simulink model "sampleModel2020_2_sub"  (R2023a)
settings: Solver=VariableStepAuto  StartTime=0.0  StopTime=10.0  RelTol=1e-3
libraries: hdlsllib x8, simulink x2
settings Model: Creator=user1  LastModifiedBy=user1

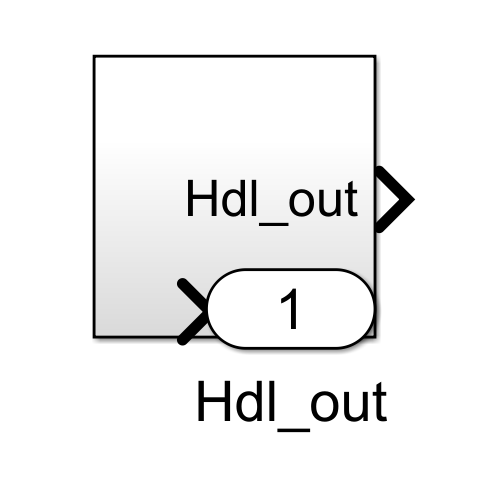
[thumbnail: Simulink's stored preview of the top-level diagram]
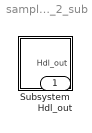
== system sampleModel2020_2_sub ==
  Subsystem : Subsystem
  Hdl_out : Outport  OutDataTypeStr=uint8

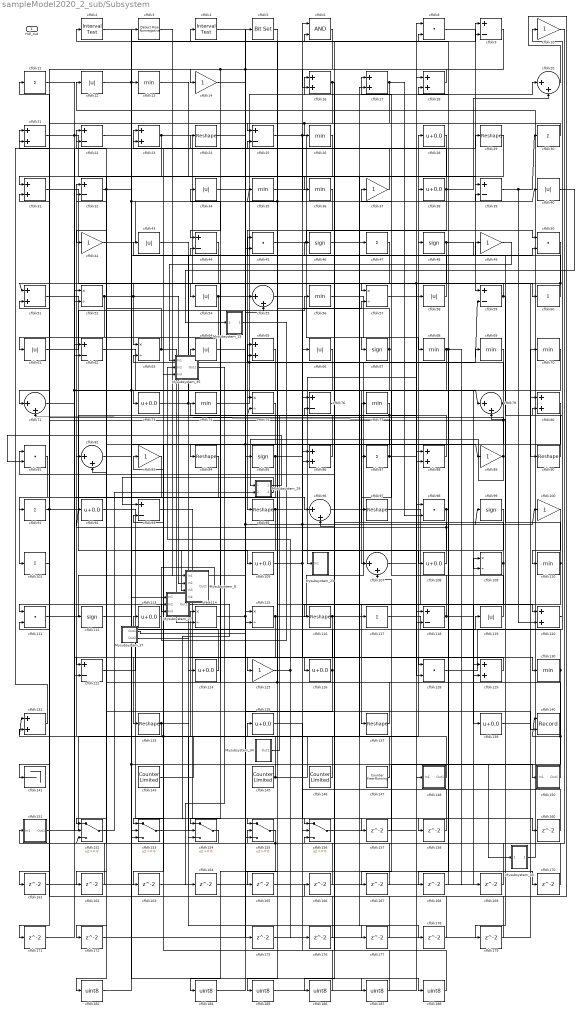
== system sampleModel2020_2_sub/Subsystem ==
  Mysubsystem_15 : Subsystem  TreatAsAtomicUnit=on  RTWFcnName=Mysubsystem_15
      settings: RTWFcnNameOpts=User specified  RTWFileNameOpts=Use function name
  Mysubsystem_23 : Subsystem  TreatAsAtomicUnit=on  RTWFcnName=Mysubsystem_23
      settings: RTWFcnNameOpts=User specified  RTWFileNameOpts=Use function name
  Mysubsystem_27 : Subsystem  TreatAsAtomicUnit=on  RTWFcnName=Mysubsystem_27
      settings: RTWFcnNameOpts=User specified  RTWFileNameOpts=Use function name
  Mysubsystem_29 : Subsystem  TreatAsAtomicUnit=on  RTWFcnName=Mysubsystem_29
      settings: RTWFcnNameOpts=User specified  RTWFileNameOpts=Use function name
  Mysubsystem_34 : Subsystem  TreatAsAtomicUnit=on  RTWFcnName=Mysubsystem_34
      settings: RTWFcnNameOpts=User specified  RTWFileNameOpts=Use function name
  Mysubsystem_35 : Subsystem  TreatAsAtomicUnit=on  RTWFcnName=Mysubsystem_35
      settings: RTWFcnNameOpts=User specified  RTWFileNameOpts=Use function name
  Mysubsystem_37 : Subsystem  TreatAsAtomicUnit=on  RTWFcnName=Mysubsystem_37
      settings: RTWFcnNameOpts=User specified  RTWFileNameOpts=Use function name
  Mysubsystem_43 : Subsystem  TreatAsAtomicUnit=on  RTWFcnName=Mysubsystem_43
      settings: RTWFcnNameOpts=User specified  RTWFileNameOpts=Use function name
  Mysubsystem_8 : Subsystem  TreatAsAtomicUnit=on  RTWFcnName=Mysubsystem_8
      settings: RTWFcnNameOpts=User specified  RTWFileNameOpts=Use function name
  cfblk{10,14,37,42,49,83,89,100,125} (9 alike) : Gain  OutDataTypeStr=uint8
  cfblk{11,30,47,60,87,91,101,117} (8 alike) : Sum  Inputs=+  OutDataTypeStr=uint8
  cfblk{28,38,73,92,105,108,113,124,126,135,139} (11 alike) : Bias  Bias=0.0  SaturateOnIntegerOverflow=off
  cfblk{20,55,71,79,82,96,107} (7 alike) : Sum  Inputs=|++  OutDataTypeStr=uint8
  cfblk{52,57,63,75,109,114..115} (7 alike) : Product  Inputs=*/  OutDataTypeStr=uint8  RndMeth=Zero  SaturateOnIntegerOverflow=on
  cfblk{13,26,35..36,56,68..70,74,77,110,130} (12 alike) : MinMax  OutDataTypeStr=uint8
  cfblk{8,45,50,81,98,111,128} (7 alike) : DotProduct  OutDataTypeStr=uint8
  cfblk{46,48,67,85,99,112} (6 alike) : Signum
  cfblk{24,29,84,90,95,97,116,133,137} (9 alike) : Reshape
  cfblk{9,22,25,32,39,44,59,62,76,93,118,122} (12 alike) : Sum  Inputs=+-  OutDataTypeStr=uint8
  cfblk{12,34,40,43,54,58,61,64,66,119} (10 alike) : Abs  OutDataTypeStr=uint8  SaturateOnIntegerOverflow=off
  cfblk{16..18,21,23,31,51,65,80,86,88,120,129,131} (14 alike) : Sum  OutDataTypeStr=uint8
  cfblk140 : Record  FileSettingsInternal="{\"entries\":[{\"content\":{\"excelSettings\":{\"content\":{},\"type\":\"Streamout.ExcelSettings\"}},\"type\":\"Streamout.FileSettingStorage\",\"uuid\":\"\"}],\"packageUris\":[\"http:\\/\\/schema.mathworks.com\\/mf0\\/streamout_blocks\\/R2020a\"],\"version\":\"1.0\"}"  Layout=[1 1]  SignalsInternal="{\"entries\":[{\"content\":{\"signals\":[{\"content\":{\"blockPath\":[],\"dimensions\":[1],\"domain\":\"\",\"lineColor\":\"#a2142f\",\"plots\":[1],\"port\":1,\"signalID\":59444,\"signalName\":\"cfblk150\"},\"type\":\"RecordBlkView.Signal\",\"uuid\":\"\"},{\"content\":{\"blockPath\":[],\"dimensions\":[1],\"domain\":\"\",\"lineColor\":\"#139fff\",\"plots\":[1],\"port\":2,\"signalID\":59447,\"signalName\":\"cfblk54\"},\"type\":\"RecordBlkView.Signal\",\"uuid\":\"\"}]},\"type\":\"RecordBlkView.InputSignals\",\"uuid\":\"\"}],\"packageUris\":[\"http:\\/\\/schema.mathworks.com\\/mf0\\/streamout_blocks\\/R2020a\"],\"version\":\"1.0\"}"  VisualizationBindings="{\"xyplotplugin\":{\"info\":[{\"series\":[{\"bindingParametersList\":[{\"parameter\":\"X-Axis\",\"signalID\":59444,\"signalName\":\"cfblk150\"},{\"parameter\":\"Y-Axis\",\"signalID\":59447,\"signalName\":\"cfblk54\"}],\"seriesID\":10474}],\"subplotID\":1}]}}"  CompatibilityTag=XY  st=-1
  cfblk141 : Terminator
  cfblk143 : hdlsllib/Sources/Counter Limited  uplimit=7  tsamp=-1
  cfblk145 : hdlsllib/Sources/Counter Limited  uplimit=7  tsamp=-1
  cfblk146 : hdlsllib/Sources/Counter Limited  uplimit=7  tsamp=-1
  cfblk147 : hdlsllib/Sources/Counter Free-Running  NumBits=16  tsamp=-1
  cfblk148 : Subsystem
      settings: LibrarySourceBlock=|
      | hdlsllib/Ports &
      | Subsystems/Subsystem
  cfblk150 : Subsystem
      settings: LibrarySourceBlock=|
      | hdlsllib/Ports &
      | Subsystems/Subsystem
  cfblk151 : Subsystem
      settings: LibrarySourceBlock=|
      | hdlsllib/Ports &
      | Subsystems/Subsystem
  cfblk{152..156} (5 alike) : Switch  OutDataTypeStr=uint8  SaturateOnIntegerOverflow=off  InputSameDT=off
  cfblk{157..158,160..172,175..179} (20 alike) : Delay  SampleTime=1
  cfblk{182,184..188} (6 alike) : DataTypeConversion  OutDataTypeStr=uint8  SaturateOnIntegerOverflow=off  RndMeth=Floor
  cfblk2 : hdlsllib/Logic and Bit Operations/Interval Test  IntervalClosedRight=on  uplimit=0.5  IntervalClosedLeft=on  lowlimit=-0.5  OutDataTypeStr=uint8
  cfblk3 : hdlsllib/Logic and Bit Operations/Detect Rise Nonnegative  vinit=0  OutDataTypeStr=uint8
  cfblk4 : hdlsllib/Logic and Bit Operations/Interval Test  IntervalClosedRight=on  uplimit=0.5  IntervalClosedLeft=on  lowlimit=-0.5  OutDataTypeStr=uint8
  cfblk5 : simulink/Logic and Bit Operations/Bit Set  iBit=0
      settings: LibrarySourceBlock=|
      | hdlsllib/Logic and Bit
      | Operations/Bit Set
  cfblk6 : Logic  AllPortsSameDT=off  OutDataTypeStr=boolean
  Hdl_out : Outport  OutDataTypeStr=uint8
  wires:
  cfblk28/1 -> cfblk31/1
  cfblk66/1 -> cfblk73/1
  cfblk44/1 -> cfblk63/1, Mysubsystem_8/2(In2)
  cfblk100/1 -> cfblk110/1
  cfblk109/1 -> cfblk81/1, cfblk137/1
  cfblk25/1 -> cfblk130/1, cfblk67/1
  cfblk98/1 -> cfblk153/3, cfblk2/1
  cfblk93/1 -> cfblk156/1
  cfblk16/1 -> cfblk126/1, cfblk125/1, cfblk26/1
  cfblk145/1 -> cfblk111/2, cfblk28/1
  cfblk150/1(Out1) -> cfblk44/2, cfblk140/1
  cfblk124/1 -> cfblk83/1
  cfblk113/1 -> cfblk111/1
  cfblk115/1 -> cfblk122/2, cfblk38/1
  cfblk146/1 -> cfblk32/1
  cfblk59/1 -> cfblk179/1, cfblk54/1
  cfblk95/1 -> cfblk120/1, Mysubsystem_8/3(In3)
  cfblk88/1 -> cfblk17/1
  cfblk56/1 -> cfblk88/2
  cfblk155/1 -> cfblk184/1, cfblk152/3
  cfblk35/1 -> cfblk68/1
  cfblk110/1 -> cfblk165/1, cfblk79/2
  cfblk51/1 -> cfblk105/1
  cfblk84/1 -> cfblk153/1
  cfblk99/1 -> cfblk116/1
  cfblk131/1 -> cfblk22/1
  cfblk70/1 -> cfblk107/1
  cfblk32/1 -> cfblk188/1, cfblk162/1
  cfblk54/1 -> cfblk140/2, cfblk61/1
  cfblk128/1 -> cfblk80/2
  cfblk23/1 -> cfblk82/2, cfblk90/1
  cfblk117/1 -> cfblk119/1
  cfblk62/1 -> cfblk109/2
  cfblk105/1 -> cfblk118/2, cfblk57/2, cfblk99/1
  cfblk74/1 -> cfblk59/2, cfblk16/1
  cfblk45/1 -> cfblk50/1, cfblk60/1
  cfblk18/1 -> cfblk14/1
  cfblk26/1 -> cfblk52/2
  cfblk147/1 -> cfblk114/1
  cfblk61/1 -> cfblk56/1
  cfblk37/1 -> cfblk23/1
  cfblk34/1 -> cfblk20/1
  cfblk92/1 -> cfblk155/1
  cfblk82/1 -> cfblk48/1
  cfblk36/1 -> cfblk95/1
  cfblk156/1 -> cfblk8/1
  cfblk10/1 -> cfblk155/2
  cfblk22/1 -> cfblk3/1
  cfblk21/1 -> cfblk96/1, cfblk117/1
  cfblk154/1 -> cfblk151/1(In1)
  cfblk24/1 -> cfblk160/1, cfblk89/1
  cfblk151/1(Out1) -> cfblk47/1
  cfblk116/1 -> cfblk178/1, cfblk133/1
  cfblk67/1 -> cfblk4/1, cfblk154/1
  cfblk60/1 -> cfblk46/1, cfblk51/1
  cfblk17/1 -> cfblk98/2, cfblk141/1
  cfblk39/1 -> cfblk120/2, cfblk30/1
  cfblk126/1 -> cfblk152/1, cfblk64/1
  cfblk77/1 -> cfblk182/1, cfblk75/2
  cfblk122/1 -> cfblk55/1
  cfblk79/1 -> cfblk96/2, cfblk34/1
  cfblk125/1 -> cfblk176/1, Mysubsystem_35/2(In2)
  cfblk14/1 -> cfblk57/1
  cfblk31/1 -> cfblk66/1
  cfblk12/1 -> cfblk13/1, cfblk187/1, Mysubsystem_43/1(In1)
  cfblk38/1 -> cfblk75/1, cfblk20/2, cfblk24/1
  cfblk96/1 -> cfblk58/1
  cfblk86/1 -> cfblk45/1
  cfblk52/1 -> cfblk62/2, Mysubsystem_27/1(In1)
  cfblk43/1 -> cfblk124/1
  cfblk8/1 -> cfblk59/1
  cfblk47/1 -> cfblk84/1
  cfblk6/1 -> cfblk155/3, cfblk171/1, cfblk44/1
  cfblk89/1 -> cfblk31/2, cfblk21/1, Mysubsystem_29/1(In1)
  cfblk97/1 -> cfblk129/1
  cfblk139/1 -> cfblk70/1
  cfblk85/1 -> cfblk87/1, cfblk101/1
  cfblk91/1 -> cfblk21/2, cfblk18/1
  cfblk130/1 -> cfblk167/1, cfblk65/1
  cfblk48/1 -> cfblk50/2, cfblk71/1, Mysubsystem_23/1(In1)
  cfblk120/1 -> cfblk10/1
  cfblk69/1 -> cfblk128/1
  cfblk118/1 -> cfblk63/2, cfblk139/1
  cfblk4/1 -> cfblk36/1
  cfblk13/1 -> cfblk39/1
  cfblk111/1 -> cfblk55/2
  cfblk65/1 -> cfblk152/2, cfblk153/2
  cfblk68/1 -> cfblk97/1, cfblk169/1, cfblk168/1
  cfblk108/1 -> cfblk92/1, cfblk77/1
  cfblk148/1(Out1) -> cfblk131/1, Mysubsystem_35/3(In3)
  cfblk101/1 -> cfblk11/1
  cfblk133/1 -> cfblk177/1, cfblk131/2
  cfblk55/1 -> cfblk108/1
  cfblk107/1 -> cfblk9/1
  cfblk81/1 -> cfblk91/1
  cfblk42/1 -> cfblk6/1
  cfblk63/1 -> cfblk114/2, cfblk32/2
  cfblk57/1 -> cfblk128/2
  cfblk112/1 -> cfblk40/1, cfblk9/2
  cfblk153/1 -> cfblk135/1
  cfblk30/1 -> cfblk25/1
  cfblk114/1 -> cfblk170/1, cfblk39/2, cfblk100/1
  cfblk90/1 -> cfblk43/1
  cfblk29/1 -> cfblk42/1
  cfblk143/1 -> cfblk17/2
  cfblk9/1 -> cfblk16/2
  cfblk58/1 -> cfblk35/1, cfblk25/2
  cfblk129/1 -> cfblk122/1
  cfblk87/1 -> cfblk69/1, cfblk71/2
  cfblk73/1 -> cfblk129/2, cfblk49/1
  cfblk2/1 -> cfblk86/2
  cfblk71/1 -> cfblk29/1
  cfblk137/1 -> cfblk65/2, cfblk22/2
  cfblk46/1 -> cfblk150/1(In1)
  cfblk11/1 -> cfblk79/1, cfblk112/1
  cfblk80/1 -> cfblk115/2, cfblk154/2
  cfblk119/1 -> cfblk37/1
  cfblk157/1 -> cfblk107/2
  cfblk135/1 -> cfblk158/1
  cfblk158/1 -> cfblk118/1
  cfblk160/1 -> cfblk86/1
  cfblk83/1 -> cfblk161/1
  cfblk161/1 -> cfblk45/2
  cfblk162/1 -> cfblk52/1
  cfblk75/1 -> cfblk163/1
  cfblk163/1 -> cfblk109/1
  cfblk164/1 -> cfblk115/1
  cfblk165/1 -> cfblk98/1
  cfblk20/1 -> cfblk166/1
  cfblk166/1 -> cfblk23/2
  cfblk167/1 -> cfblk82/1
  cfblk168/1 -> cfblk8/2
  cfblk169/1 -> cfblk6/2
  cfblk170/1 -> cfblk18/2
  cfblk171/1 -> cfblk62/1
  cfblk50/1 -> cfblk172/1
  cfblk172/1 -> cfblk80/1
  cfblk64/1 -> cfblk175/1
  cfblk175/1 -> cfblk88/1
  cfblk176/1 -> cfblk51/2
  cfblk177/1 -> cfblk93/2
  cfblk178/1 -> cfblk156/3
  cfblk179/1 -> cfblk156/2
  cfblk184/1 -> cfblk5/1
  cfblk5/1 -> cfblk185/1
  cfblk185/1 -> cfblk148/1(In1)
  cfblk76/1 -> cfblk186/1
  cfblk186/1 -> cfblk113/1
  cfblk187/1 -> cfblk76/1
  cfblk188/1 -> cfblk76/2
  cfblk3/1 -> Mysubsystem_8/1(In1)
  cfblk182/1 -> Mysubsystem_8/4(In4)
  cfblk40/1 -> Mysubsystem_15/1(In1)
  Mysubsystem_15/1(Out1) -> Mysubsystem_27/2(In2)
  Mysubsystem_8/1(Out1) -> Mysubsystem_27/3(In3)
  Mysubsystem_27/1(Out1) -> cfblk157/1
  cfblk152/1 -> Mysubsystem_29/2(In2)
  Mysubsystem_29/1(y) -> cfblk81/2
  Mysubsystem_29/2(Out2) -> cfblk93/1
  Mysubsystem_34/1(Out1) -> cfblk74/1
  cfblk49/1 -> Mysubsystem_35/1(In1)
  Mysubsystem_35/1(Out1) -> cfblk164/1
  Mysubsystem_37/1(Out1) -> cfblk85/1
  Mysubsystem_37/2(Out2) -> cfblk154/3
  Mysubsystem_43/1(Out1) -> cfblk12/1

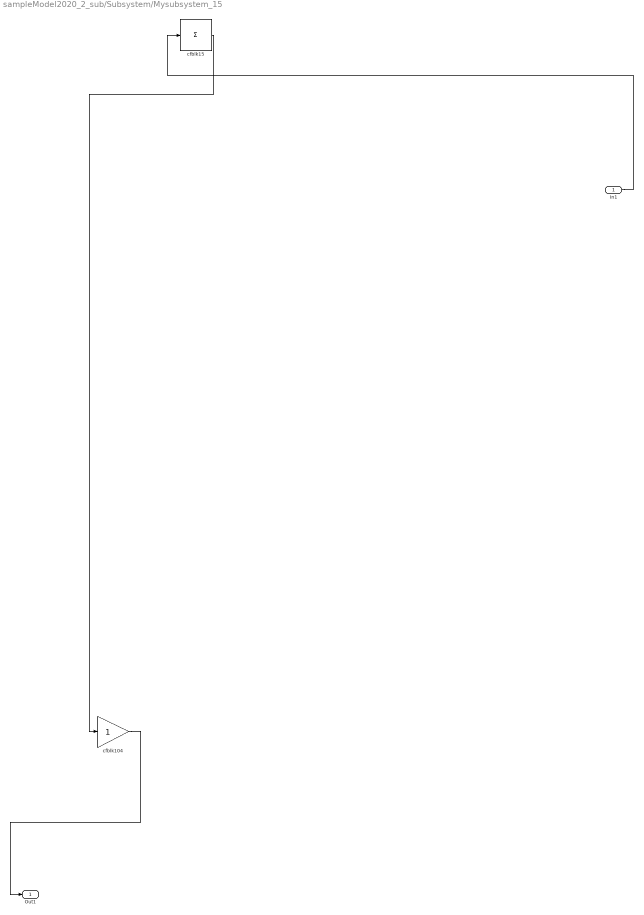
== system sampleModel2020_2_sub/Subsystem/Mysubsystem_15 ==
  In1 : Inport
  cfblk104 : Gain
  cfblk15 : Sum  Inputs=+
  Out1 : Outport
  wires:
  In1/1 -> cfblk15/1
  cfblk104/1 -> Out1/1
  cfblk15/1 -> cfblk104/1

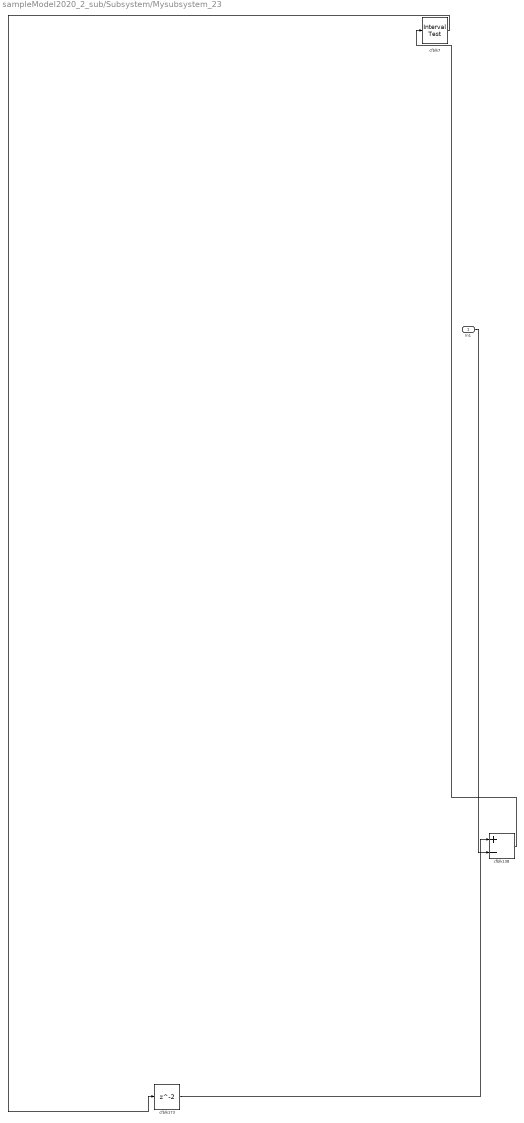
== system sampleModel2020_2_sub/Subsystem/Mysubsystem_23 ==
  In1 : Inport
  cfblk138 : Sum  Inputs=+-
  cfblk173 : Delay  SampleTime=1
  cfblk7 : hdlsllib/Logic and Bit Operations/Interval Test  IntervalClosedRight=on  uplimit=0.5  IntervalClosedLeft=on  lowlimit=-0.5  OutDataTypeStr=boolean
  wires:
  In1/1 -> cfblk138/2
  cfblk7/1 -> cfblk173/1
  cfblk173/1 -> cfblk138/1
  cfblk138/1 -> cfblk7/1

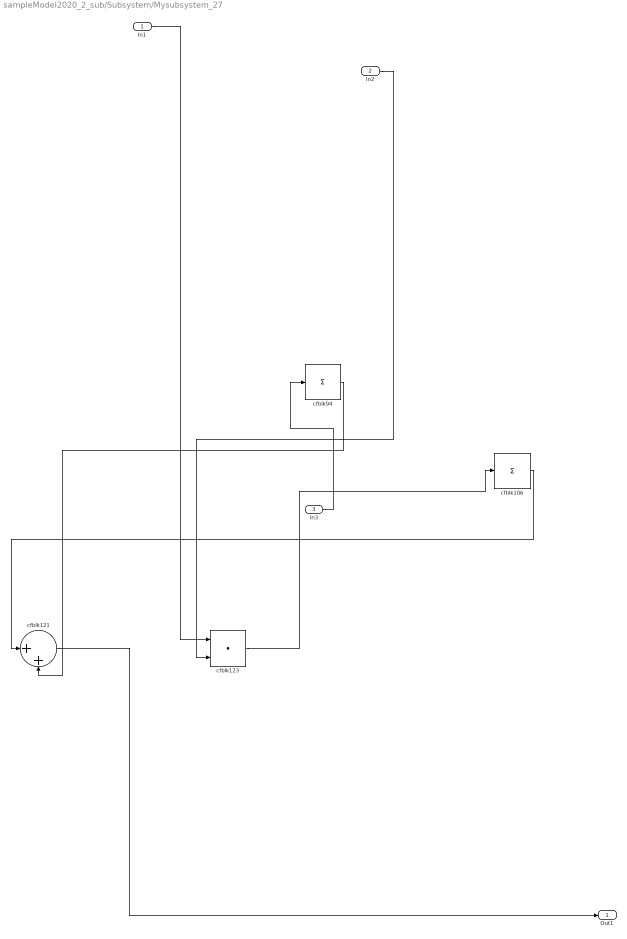
== system sampleModel2020_2_sub/Subsystem/Mysubsystem_27 ==
  In1 : Inport
  In2 : Inport  Port=2
  In3 : Inport  Port=3
  cfblk106 : Sum  Inputs=+
  cfblk121 : Sum  Inputs=|++
  cfblk123 : DotProduct  OutDataTypeStr=Inherit: Inherit via internal rule
  cfblk94 : Sum  Inputs=+
  Out1 : Outport
  wires:
  In2/1 -> cfblk123/2
  cfblk94/1 -> cfblk121/2
  cfblk106/1 -> cfblk121/1
  In1/1 -> cfblk123/1
  In3/1 -> cfblk94/1
  cfblk123/1 -> cfblk106/1
  cfblk121/1 -> Out1/1

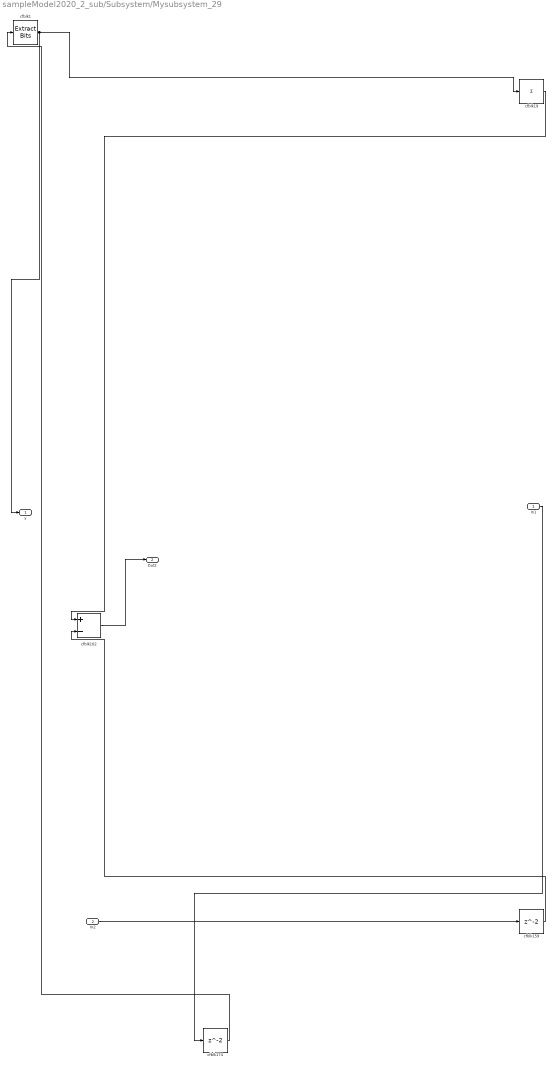
== system sampleModel2020_2_sub/Subsystem/Mysubsystem_29 ==
  In1 : Inport
  In2 : Inport  Port=2
  cfblk1 : simulink/Logic and Bit Operations/Extract Bits  bitsToExtract=Upper half  numBits=8  bitIdxRange=[0 7]  outScalingMode=Preserve fixed-point scaling
      settings: LibrarySourceBlock=|
      | hdlsllib/Logic and Bit
      | Operations/Extract Bits
  cfblk102 : Sum  Inputs=+-
  cfblk159 : Delay  SampleTime=1
  cfblk174 : Delay  SampleTime=1
  cfblk19 : Sum  Inputs=+
  y : Outport
  Out2 : Outport  Port=2
  wires:
  cfblk174/1 -> cfblk1/1
  cfblk159/1 -> cfblk102/2
  cfblk1/1 -> cfblk19/1, y/1
  In2/1 -> cfblk159/1
  cfblk19/1 -> cfblk102/1
  In1/1 -> cfblk174/1
  cfblk102/1 -> Out2/1

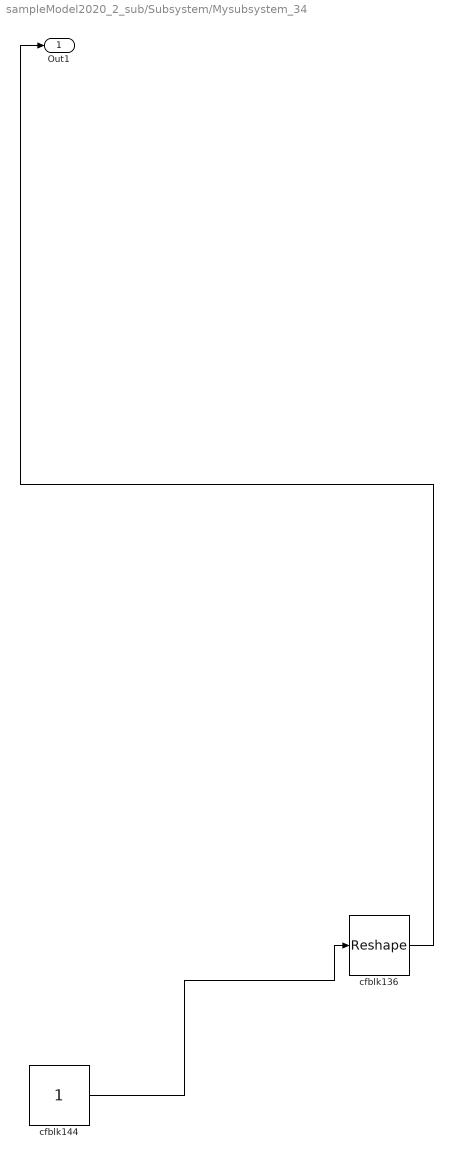
== system sampleModel2020_2_sub/Subsystem/Mysubsystem_34 ==
  cfblk136 : Reshape
  cfblk144 : Constant  SampleTime=-1
  Out1 : Outport
  wires:
  cfblk136/1 -> Out1/1
  cfblk144/1 -> cfblk136/1

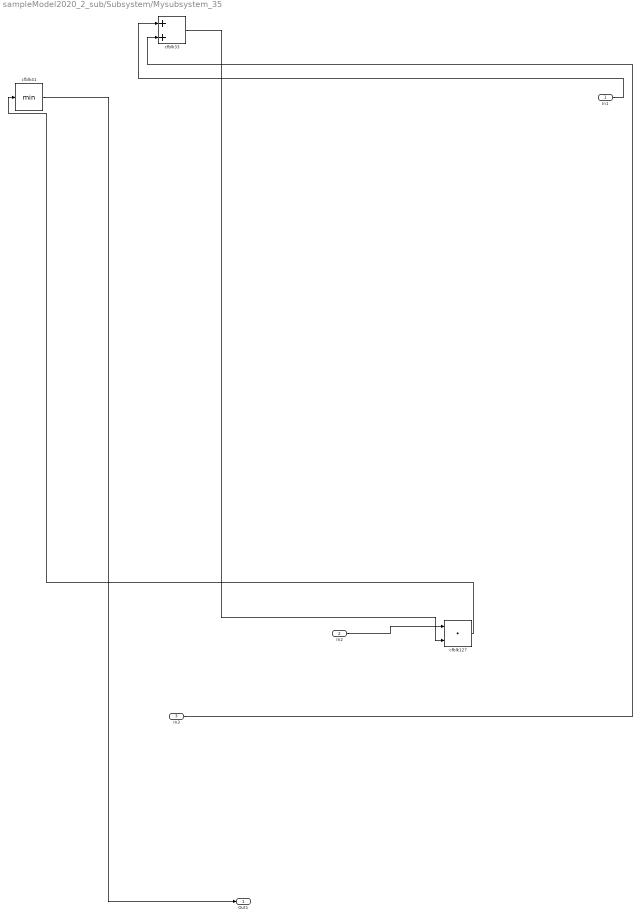
== system sampleModel2020_2_sub/Subsystem/Mysubsystem_35 ==
  In1 : Inport
  In2 : Inport  Port=2
  In3 : Inport  Port=3
  cfblk127 : DotProduct  OutDataTypeStr=Inherit: Inherit via internal rule
  cfblk33 : Sum
  cfblk41 : MinMax
  Out1 : Outport
  wires:
  In2/1 -> cfblk127/1
  In1/1 -> cfblk33/1
  In3/1 -> cfblk33/2
  cfblk41/1 -> Out1/1
  cfblk33/1 -> cfblk127/2
  cfblk127/1 -> cfblk41/1

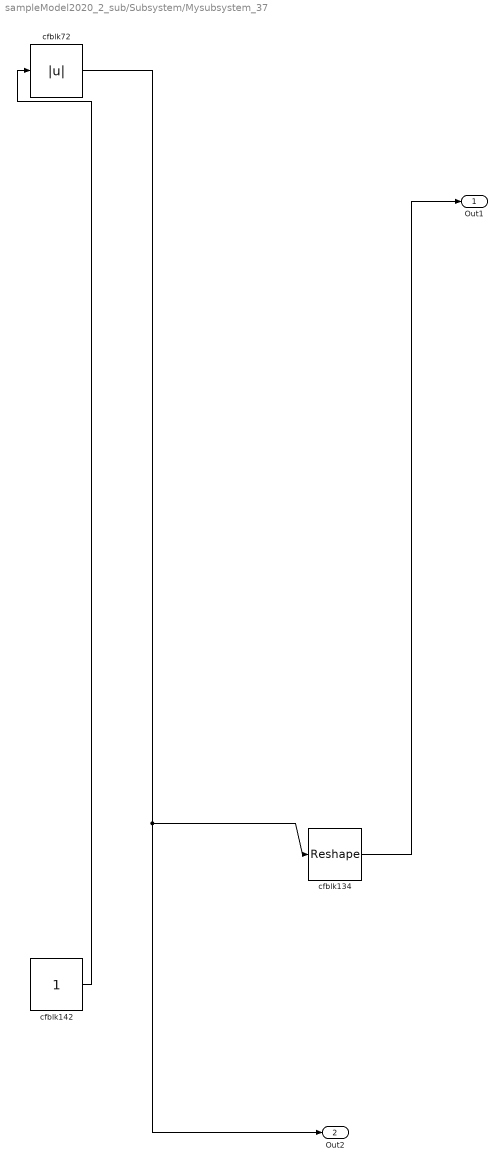
== system sampleModel2020_2_sub/Subsystem/Mysubsystem_37 ==
  cfblk134 : Reshape
  cfblk142 : Constant  SampleTime=-1
  cfblk72 : Abs  SaturateOnIntegerOverflow=off
  Out1 : Outport
  Out2 : Outport  Port=2
  wires:
  cfblk134/1 -> Out1/1
  cfblk142/1 -> cfblk72/1
  cfblk72/1 -> cfblk134/1, Out2/1

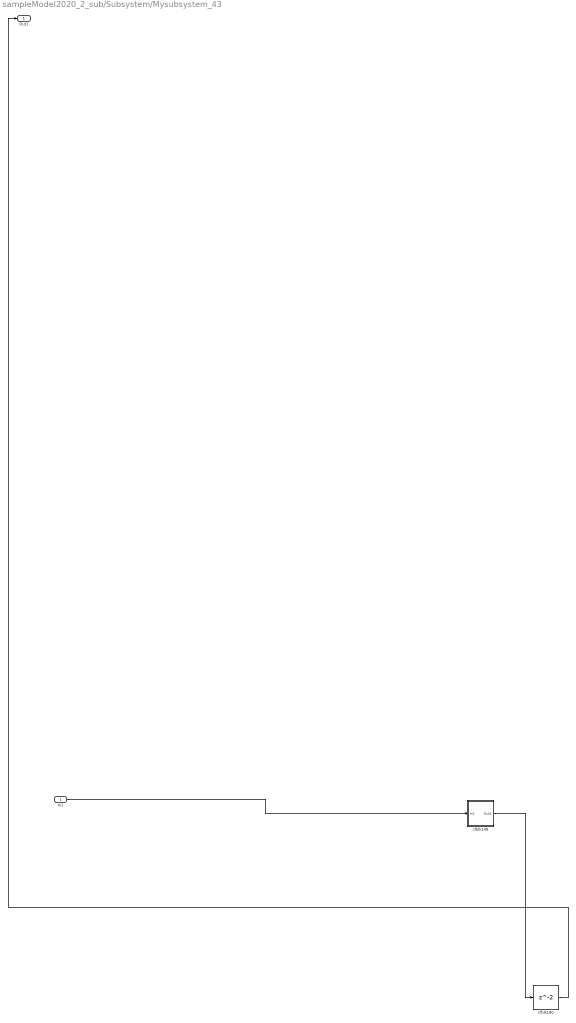
== system sampleModel2020_2_sub/Subsystem/Mysubsystem_43 ==
  In1 : Inport
  cfblk149 : Subsystem
      settings: LibrarySourceBlock=|
      | hdlsllib/Ports &
      | Subsystems/Subsystem
  cfblk180 : Delay  SampleTime=1
  Out1 : Outport
  wires:
  In1/1 -> cfblk149/1(In1)
  cfblk180/1 -> Out1/1
  cfblk149/1(Out1) -> cfblk180/1

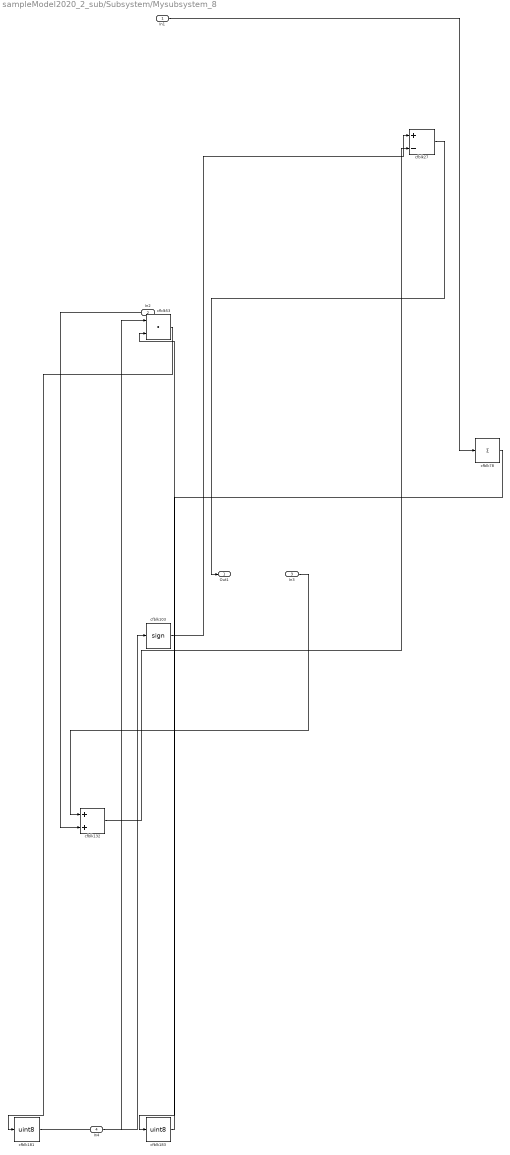
== system sampleModel2020_2_sub/Subsystem/Mysubsystem_8 ==
  In1 : Inport
  In2 : Inport  Port=2
  In3 : Inport  Port=3
  In4 : Inport  Port=4
  cfblk103 : Signum
  cfblk132 : Sum
  cfblk181 : DataTypeConversion  OutDataTypeStr=uint8  SaturateOnIntegerOverflow=off  RndMeth=Floor
  cfblk183 : DataTypeConversion  OutDataTypeStr=uint8  SaturateOnIntegerOverflow=off  RndMeth=Floor
  cfblk27 : Sum  Inputs=+-
  cfblk53 : DotProduct  OutDataTypeStr=Inherit: Inherit via internal rule
  cfblk78 : Sum  Inputs=+
  Out1 : Outport
  wires:
  In4/1 -> cfblk53/1
  In1/1 -> cfblk78/1
  cfblk27/1 -> Out1/1
  cfblk53/1 -> cfblk181/1
  cfblk183/1 -> cfblk53/2
  cfblk181/1 -> cfblk103/1
  cfblk78/1 -> cfblk183/1
  In3/1 -> cfblk132/1
  cfblk132/1 -> cfblk27/2
  In2/1 -> cfblk132/2
  cfblk103/1 -> cfblk27/1

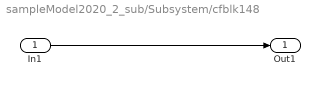
== system sampleModel2020_2_sub/Subsystem/cfblk148 ==
  In1 : Inport
  Out1 : Outport
  wires:
  In1/1 -> Out1/1

== system sampleModel2020_2_sub/Subsystem/cfblk150 ==
  In1 : Inport
  Out1 : Outport
  wires:
  In1/1 -> Out1/1

== system sampleModel2020_2_sub/Subsystem/cfblk151 ==
  In1 : Inport
  Out1 : Outport
  wires:
  In1/1 -> Out1/1

== system sampleModel2020_2_sub/Subsystem/Mysubsystem_43/cfblk149 ==
  In1 : Inport
  Out1 : Outport
  wires:
  In1/1 -> Out1/1
